simulink model "Maglev_LMPC"  (R2023b)
settings: Solver=VariableStepAuto  StartTime=0.0  StopTime=1  RelTol=1e-3
values from neighbouring files (symbols this model uses):
  A_ob = A - L*C    [main_LMPC.m]
  B_ob = [ B - L*D, L]    [main_LMPC.m]
  C_ob = eye(n)    [main_LMPC.m]
  D_ob = zeros(n, m+p)    [main_LMPC.m]
undefined symbols (not defined in the file or in its folder): x1_eq0, x2_eq0
settings Model: Creator=fabio  LastModifiedBy=lollo
settings SolverCC: AlgebraicLoopSolver=TrustRegion
settings OptimizationCC: BlockReduction=off  DefaultParameterBehavior=Inlined  BufferReuse=off  ReuseModelBlockBuffer=off
settings DebuggingCC: UnconnectedInputMsg=warning  UnconnectedOutputMsg=warning  UnconnectedLineMsg=warning
settings ModelReferenceCC: EnableRefExpFcnMdlSchedulingChecks=on
settings RTWCC: DLArmComputeVersion=19.05

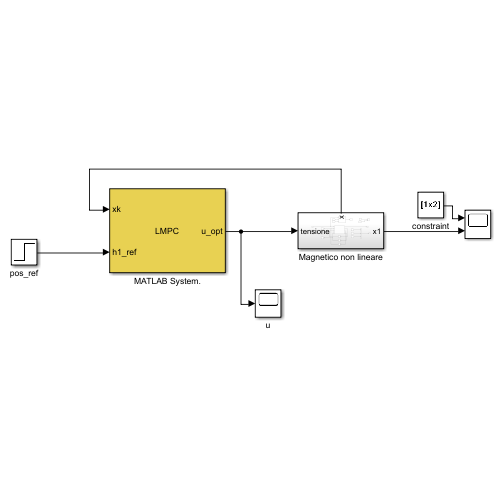
[thumbnail: Simulink's stored preview of the top-level diagram]
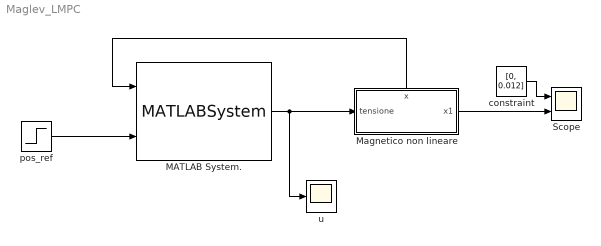
== system Maglev_LMPC ==
  MATLAB System. : MATLABSystem  System=LMPC  N=10  Q=1  R=1  tau_s=0.02  SimulateUsing=Interpreted execution
      mask Type: LMPC
      mask Display:
      | disp('LMPC');
      | port_label('input',1,'xk');
      | port_label('input',2,'h1_ref');
      | port_label('output',1,'u_opt');
  Magnetico non lineare : Subsystem
      settings: PortSchema="{\"entries\":[{\"content\":{\"sides\":[{\"content\":{\"connectorIds\":[\"In1\"]},\"type\":\"ConnectorPlacement.EquallySpacedRectSide\",\"uuid\":\"4c2628b7-19c4-4753-accd-078547eff280\"},{\"content\":{\"connectorIds\":[\"Out1\"],\"side\":\"RIGHT\"},\"type\":\"ConnectorPlacement.EquallySpacedRectSide\",\"uuid\":\"46f8a782-99b4-4db5-ac9e-879226864e1a\"},{\"content\":{\"connectorIds\":[\"Out2\"],\"side\":\"TOP\"},\"type\":\"ConnectorPlacement.EquallySpacedRectSide\",\"uuid\":\"e9ea6a3a-0b10-4f27-be26-5b91ce6de957\"}]},\"type\":\"ConnectorPlacement.EquallySpacedConnector\",\"uuid\":\"8380a659-82e1-48e4-be7e-4b84feeb9f50\"}],\"packageUris\":[\"http://schema.mathworks.com/mf0/Connector/R2020b\"],\"version\":\"1.0\"}"
  Scope : Scope  NumInputPorts=2
  constraint : Constant  Value=[0, 0.012]
  pos_ref : Step  Time=0  After=0.004  SampleTime=0
  u : Scope
  wires:
  pos_ref/1 -> MATLAB System./2
  MATLAB System./1 -> Magnetico non lineare/1(tensione), u/1
  Magnetico non lineare/2(x) -> MATLAB System./1
  Magnetico non lineare/1(x1) -> Scope/2
  constraint/1 -> Scope/1

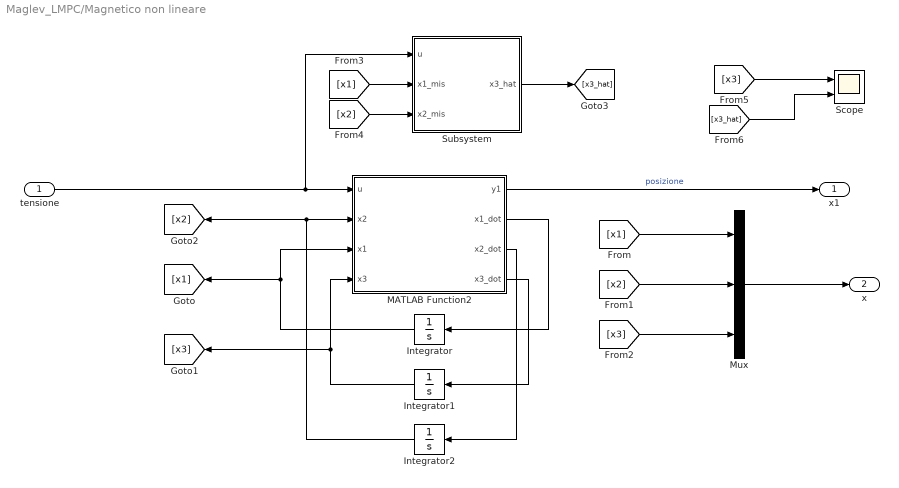
== system Maglev_LMPC/Magnetico non lineare ==
  tensione : Inport
  Integrator : Integrator
  Integrator1 : Integrator
  Integrator2 : Integrator
  MATLAB Function2 : MATLAB Function  TreatAsAtomicUnit=on
  Mux : Mux  Inputs=3
  Scope : Scope  NumInputPorts=2
  Subsystem : Subsystem
  x1 : Outport
  x : Outport  Port=2
  wires:
  tensione/1 -> Subsystem/1(u), MATLAB Function2/1(u)
  MATLAB Function2/1(y1) -> x1/1  "posizione"
  MATLAB Function2/2(x1_dot) -> Integrator/1
  Integrator/1 -> MATLAB Function2/3(x1), [x1]
  MATLAB Function2/4(x3_dot) -> Integrator1/1
  Integrator1/1 -> [x3], MATLAB Function2/4(x3)
  [x1] -> Mux/1
  [x2] -> Mux/2
  [x3] -> Mux/3
  Mux/1 -> x/1
  MATLAB Function2/3(x2_dot) -> Integrator2/1
  Integrator2/1 -> MATLAB Function2/2(x2), [x2]
  [x1] -> Subsystem/2(x1_mis)
  [x2] -> Subsystem/3(x2_mis)
  Subsystem/1(x3_hat) -> [x3_hat]
  [x3_hat] -> Scope/2
  [x3] -> Scope/1

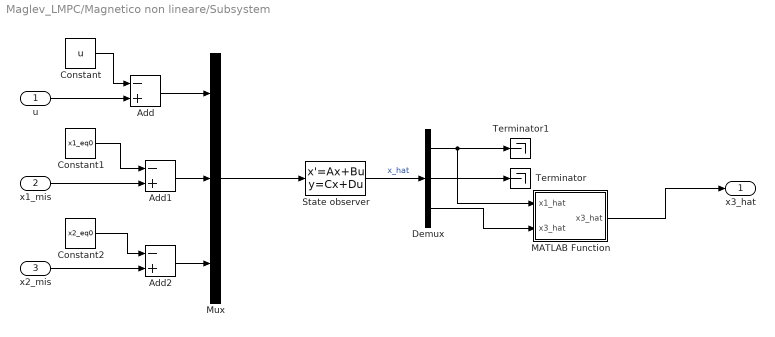
== system Maglev_LMPC/Magnetico non lineare/Subsystem ==
  u : Inport
  x1_mis : Inport  Port=2
  x2_mis : Inport  Port=3
  Add : Sum  Inputs=-+
  Add1 : Sum  Inputs=-+
  Add2 : Sum  Inputs=-+
  Constant : Constant  Value=u
  Constant1 : Constant  Value=x1_eq0
  Constant2 : Constant  Value=x2_eq0
  Demux : Demux  Outputs=3
  MATLAB Function : MATLAB Function  TreatAsAtomicUnit=on
  Mux : Mux  Inputs=3
  State observer : StateSpace  A=A_ob  B=B_ob  C=C_ob  D=D_ob  InitialCondition=[0;0;0]  ParameterTunability=Unconstrained
  Terminator : Terminator
  Terminator1 : Terminator
  x3_hat : Outport
  wires:
  x1_mis/1 -> Add1/2
  u/1 -> Add/2
  Mux/1 -> State observer/1
  State observer/1 -> Demux/1  "x_hat"
  Demux/1 -> MATLAB Function/1(x1_hat), Terminator1/1
  Demux/2 -> Terminator/1
  Constant/1 -> Add/1
  Constant1/1 -> Add1/1
  Constant2/1 -> Add2/1
  x2_mis/1 -> Add2/2
  Add/1 -> Mux/1
  Add1/1 -> Mux/2
  Add2/1 -> Mux/3
  MATLAB Function/1(x3_hat) -> x3_hat/1
  Demux/3 -> MATLAB Function/2("x3_hat ")

== matlab function Maglev_LMPC/Magnetico non lineare/Subsystem/MATLAB Function ==
  data: x1_hat input; x3_hat output; x3_hat input
function x3_hat = fcn(x1_hat, x3_hat)

if x1_hat<=0 && x3_hat<=0
    x3_hat=0;
end

== matlab function Maglev_LMPC/Magnetico non lineare/MATLAB Function2 ==
  data: u input; y1 output; x2 input; x1_dot output; x2_dot output; x1 input; x3 input; x3_dot output
function [y1,x1_dot, x2_dot, x3_dot] = fcn(u, x2, x1, x3)
    m = 0.0657;
    g = 9.81;
    k_mag = 2.4405e-05;
    Rtot = 9.7585;
    Lc = 0.3708;
    y0 = 0.012;
    
    x2_dot = 1/Lc*(-Rtot*x2 + u);

    x1_dot = x3;
    if x1 < y0
        x3_dot = (k_mag/m)*(x2/(y0-x1))^2 - g;
    else
        x1 = 0.012;
        x3_dot = 0;
        x3 = 0;
    end

    
    % condizioni
    if x1 <=0 && x3_dot < 0
        x1 = 0;
        x3 = 0;
        x3_dot = 0;
    end
y1 = x1;
